simulink model "QuantizedFullStateFeedbackSimulation"  (R2018b)
settings: Solver=VariableStepAuto  StartTime=0.0  StopTime=30  RelTol=1e-3
values from neighbouring files (symbols this model uses):
  d = 80    [GenPendulumParams.m]
  h = 0.1    [GenPendulumParams.m]
  K = place(linsyspendulum.A, linsyspendulum.B, poles)    [LinearizePendulumRCSPlant.m]
  tau = 0.101    [GenPendulumParams.m]
settings Model: Creator=mendicantbias  LastModifiedBy=mendicantbias
settings ModelReferenceCC: ModelReferenceMinAlgLoopOccurrences=on

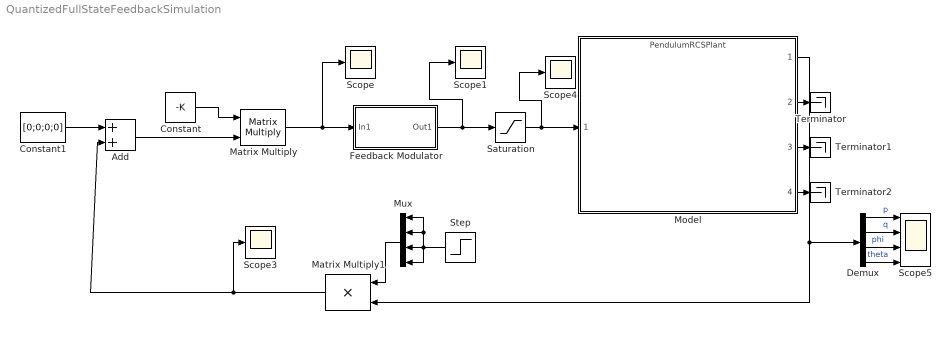
== system QuantizedFullStateFeedbackSimulation ==
  Add : Sum
  Constant : Constant  Value=-K
  Constant1 : Constant  Value=[0;0;0;0]
  Demux : Demux
  Feedback Modulator : Subsystem
  Matrix Multiply : Product  Multiplication=Matrix(*)
  Matrix Multiply1 : Product
  Model : ModelReference  ModelNameDialog=PendulumRCSPlant  SimulationMode=Normal  ModelReferenceVersion=1.183
  Mux : Mux
  Saturation : Saturate  UpperLimit=d  LowerLimit=-d
  Scope{,1,3..4} (4 alike) : Scope
  Scope5 : Scope  NumInputPorts=4
  Step : Step  Time=5  SampleTime=0
  Terminator : Terminator
  Terminator1 : Terminator
  Terminator2 : Terminator
  wires:
  Constant/1 -> Matrix Multiply/1
  Matrix Multiply/1 -> Feedback Modulator/1(In1), Scope/1
  Feedback Modulator/1(Out1) -> Saturation/1, Scope1/1
  Add/1 -> Matrix Multiply/2
  Constant1/1 -> Add/1
  Mux/1 -> Matrix Multiply1/1
  Step/1 -> Mux/3, Mux/2, Mux/1, Mux/4
  Model/2 -> Terminator/1
  Model/3 -> Terminator1/1
  Model/4 -> Terminator2/1
  Matrix Multiply1/1 -> Add/2, Scope3/1
  Demux/4 -> Scope5/4  "theta"
  Demux/2 -> Scope5/2  "q"
  Model/1 -> Matrix Multiply1/2, Demux/1
  Demux/1 -> Scope5/1  "p"
  Demux/3 -> Scope5/3  "phi"
  Saturation/1 -> Scope4/1, Model/1

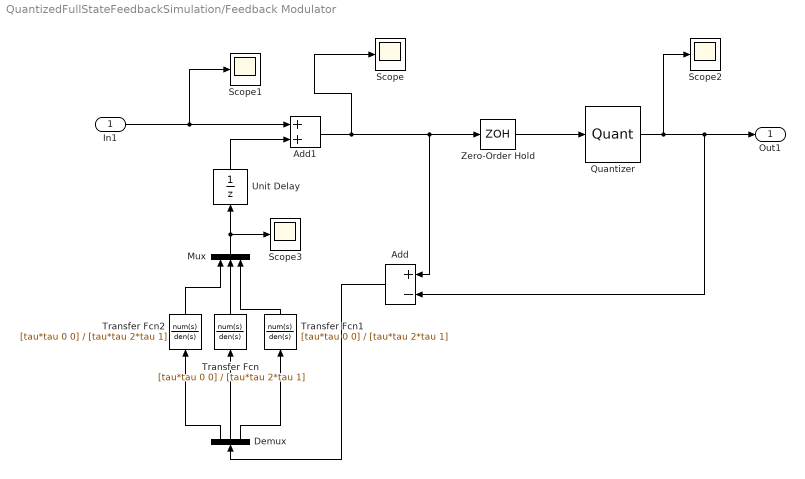
== system QuantizedFullStateFeedbackSimulation/Feedback Modulator ==
  In1 : Inport
  Add : Sum  Inputs=+-
  Add1 : Sum
  Demux : Demux  Outputs=3
  Mux : Mux  Inputs=3
  Quantizer : Quantizer  QuantizationInterval=d
  Scope{,1..3} (4 alike) : Scope
  Transfer Fcn : TransferFcn  Numerator=[tau*tau 0 0]  Denominator=[tau*tau 2*tau 1]
  Transfer Fcn1 : TransferFcn  Numerator=[tau*tau 0 0]  Denominator=[tau*tau 2*tau 1]
  Transfer Fcn2 : TransferFcn  Numerator=[tau*tau 0 0]  Denominator=[tau*tau 2*tau 1]
  Unit Delay : UnitDelay  SampleTime=-1
  Zero-Order Hold : ZeroOrderHold  SampleTime=h
  Out1 : Outport
  wires:
  Mux/1 -> Unit Delay/1, Scope3/1
  Add1/1 -> Scope/1, Zero-Order Hold/1, Add/1
  In1/1 -> Scope1/1, Add1/1
  Quantizer/1 -> Scope2/1, Out1/1, Add/2
  Zero-Order Hold/1 -> Quantizer/1
  Add/1 -> Demux/1
  Transfer Fcn/1 -> Mux/2
  Transfer Fcn2/1 -> Mux/1
  Transfer Fcn1/1 -> Mux/3
  Demux/2 -> Transfer Fcn/1
  Demux/1 -> Transfer Fcn2/1
  Demux/3 -> Transfer Fcn1/1
  Unit Delay/1 -> Add1/2
